simulink library "DYN_2018b"  (Simulink 9.2)
settings: Solver=ode45  StartTime=0.0  StopTime=10.0  RelTol=1e-3  EnableMultiTasking=on
libraries: DYN_AERO x1, DYN_ATT x1, DYN_ECLIPSE x1, DYN_EPHEM x1, DYN_GRAV x1, DYN_MAG x1, DYN_MCI x1, DYN_SRP x1, DYN_TIME x1, DYN_TRA x1
settings Model: Creator=alger  LastModifiedBy=Mike

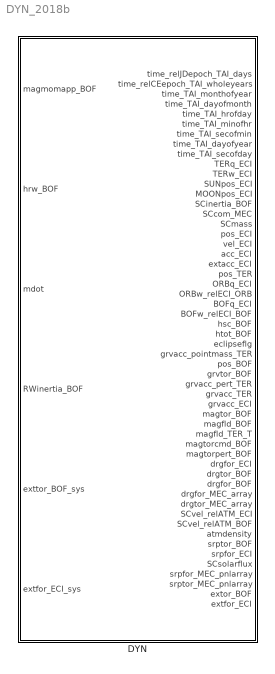
== system DYN_2018b ==
  DYN : Subsystem

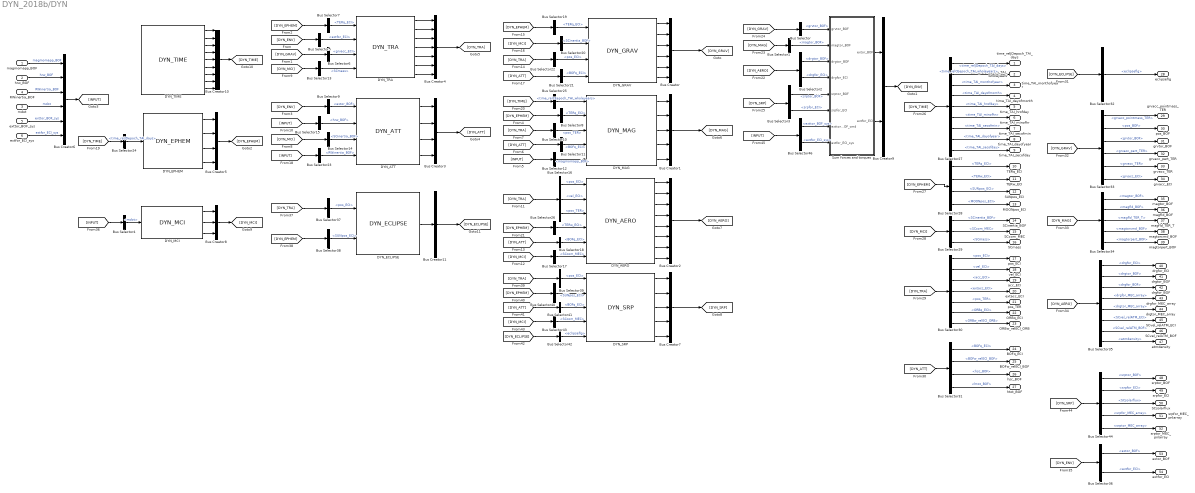
== system DYN_2018b/DYN ==
  magmomapp_BOF : Inport  PortDimensions=3
  hrw_BOF : Inport  Port=2  PortDimensions=3
  mdot : Inport  Port=3  PortDimensions=1
  RWinertia_BOF : Inport  Port=4  PortDimensions=[3,3]
  exttor_BOF_sys : Inport  Port=5  PortDimensions=3
  extfor_ECI_sys : Inport  Port=6  PortDimensions=3
  Bus Creator : BusCreator  Inputs=6
  Bus Creator1 : BusCreator  Inputs=5
  Bus Creator10 : BusCreator  Inputs=9
  Bus Creator11 : BusCreator  Inputs=1
  Bus Creator2 : BusCreator  Inputs=8
  Bus Creator3 : BusCreator  Inputs=4
  Bus Creator4 : BusCreator  Inputs=7
  Bus Creator5 : BusCreator  Inputs=4
  Bus Creator6 : BusCreator  Inputs=6
  Bus Creator7 : BusCreator  Inputs=5
  Bus Creator8 : BusCreator  Inputs=3
  Bus Creator9 : BusCreator  Inputs=2
  Bus Selector : BusSelector  OutputSignals=grvtor_BOF
  Bus Selector1 : BusSelector  OutputSignals=magtor_BOF
  Bus Selector10 : BusSelector  OutputSignals=pos_TER
  Bus Selector{11,18,21,41} (4 alike) : BusSelector  OutputSignals=BOFq_ECI
  Bus Selector12 : BusSelector  OutputSignals=magmomapp_BOF
  Bus Selector13 : BusSelector  OutputSignals=SCmass
  Bus Selector14 : BusSelector  OutputSignals=SCinertia_BOF
  Bus Selector15 : BusSelector  OutputSignals=hrw_BOF
  Bus Selector16 : BusSelector  OutputSignals=pos_ECI,vel_ECI,pos_TER
  Bus Selector17 : BusSelector  OutputSignals=SCcom_MEC
  Bus Selector19 : BusSelector  OutputSignals=TERq_ECI
  Bus Selector2 : BusSelector  OutputSignals=drgtor_BOF,drgfor_ECI
  Bus Selector20 : BusSelector  OutputSignals=SCinertia_BOF
  Bus Selector22 : BusSelector  OutputSignals=pos_ECI
  Bus Selector23 : BusSelector  OutputSignals=RWinertia_BOF
  Bus Selector24 : BusSelector  OutputSignals=time_relJDepoch_TAI_days
  Bus Selector25 : BusSelector  OutputSignals=time_relCEepoch_TAI_wholeyears
  Bus Selector26 : BusSelector  OutputSignals=TERw_ECI
  Bus Selector27 : BusSelector  OutputSignals=time_relJDepoch_TAI_days,time_relCEepoch_TAI_wholeyears,time_TAI_monthofyear,time_TAI_dayofmonth,time_TAI_hrofday,time_TAI_minofhr,time_TAI_secofmin,time_TAI_dayofyear,time_TAI_secofday
  Bus Selector28 : BusSelector  OutputSignals=TERq_ECI,TERw_ECI,SUNpos_ECI,MOONpos_ECI
  Bus Selector29 : BusSelector  OutputSignals=SCinertia_BOF,SCcom_MEC,SCmass
  Bus Selector3 : BusSelector  OutputSignals=srptor_BOF,srpfor_ECI
  Bus Selector30 : BusSelector  OutputSignals=pos_ECI,vel_ECI,acc_ECI,extacc_ECI,pos_TER,ORBq_ECI,ORBw_relECI_ORB
  Bus Selector31 : BusSelector  OutputSignals=BOFq_ECI,BOFw_relECI_BOF,hsc_BOF,htot_BOF
  Bus Selector32 : BusSelector  OutputSignals=eclipseflg
  Bus Selector33 : BusSelector  OutputSignals=grvacc_pointmass_TER,pos_BOF,grvtor_BOF,grvacc_pert_TER,grvacc_TER,grvacc_ECI
  Bus Selector34 : BusSelector  OutputSignals=magtor_BOF,magfld_BOF,magfld_TER_T,magtorcmd_BOF,magtorpert_BOF
  Bus Selector35 : BusSelector  OutputSignals=drgfor_ECI,drgtor_BOF,drgfor_BOF,drgfor_MEC_array,drgtor_MEC_array,SCvel_relATM_ECI,SCvel_relATM_BOF,atmdensity
  Bus Selector36 : BusSelector  OutputSignals=extor_BOF,extfor_ECI
  Bus Selector37 : BusSelector  OutputSignals=pos_ECI
  Bus Selector38 : BusSelector  OutputSignals=SUNpos_ECI
  Bus Selector39 : BusSelector  OutputSignals=pos_ECI
  Bus Selector4 : BusSelector  OutputSignals=mdot
  Bus Selector40 : BusSelector  OutputSignals=SUNpos_ECI
  Bus Selector42 : BusSelector  OutputSignals=eclipseflg
  Bus Selector43 : BusSelector  OutputSignals=SCcom_MEC
  Bus Selector44 : BusSelector  OutputSignals=srptor_BOF,srpfor_ECI,SCsolarflux,srpfor_MEC_array,srptor_MEC_array
  Bus Selector46 : BusSelector  OutputSignals=exttor_BOF_sys,extfor_ECI_sys
  Bus Selector5 : BusSelector  OutputSignals=extfor_ECI
  Bus Selector6 : BusSelector  OutputSignals=grvacc_ECI
  Bus Selector7 : BusSelector  OutputSignals=TERq_ECI
  Bus Selector8 : BusSelector  OutputSignals=TERq_ECI
  Bus Selector9 : BusSelector  OutputSignals=extor_BOF
  DYN_AERO : DYN_AERO/DYN_AERO  SystemSampleTime=-1  Latency=0  AutoFrameSizeCalculation=off
  DYN_ATT : DYN_ATT/DYN_ATT  SystemSampleTime=-1  Latency=0  AutoFrameSizeCalculation=off
  DYN_ECLIPSE : DYN_ECLIPSE/DYN_ECLIPSE  SystemSampleTime=-1  Latency=0  AutoFrameSizeCalculation=off
  DYN_EPHEM : DYN_EPHEM/DYN_EPHEM  SystemSampleTime=-1  Latency=0  AutoFrameSizeCalculation=off
  DYN_GRAV : DYN_GRAV/DYN_GRAV  SystemSampleTime=-1  Latency=0  AutoFrameSizeCalculation=off
  DYN_MAG : DYN_MAG/DYN_MAG  SystemSampleTime=-1  Latency=0  AutoFrameSizeCalculation=off
  DYN_MCI : DYN_MCI/DYN_MCI  SystemSampleTime=-1  Latency=0  AutoFrameSizeCalculation=off
  DYN_SRP : DYN_SRP/DYN_SRP  SystemSampleTime=-1  Latency=0  AutoFrameSizeCalculation=off
  DYN_TIME : DYN_TIME/DYN_TIME  SystemSampleTime=-1  Latency=0  AutoFrameSizeCalculation=off
  "DYN_TRA " : DYN_TRA/DYN_TRA   SystemSampleTime=-1  Latency=0  AutoFrameSizeCalculation=off
  Sum forces and torques : Subsystem
  time_relJDepoch_TAI_days : Outport  VectorParamsAs1DForOutWhenUnconnected=off
  time_relCEepoch_TAI_wholeyears : Outport  Port=2  VectorParamsAs1DForOutWhenUnconnected=off
  time_TAI_monthofyear : Outport  Port=3  VectorParamsAs1DForOutWhenUnconnected=off
  time_TAI_dayofmonth : Outport  Port=4  VectorParamsAs1DForOutWhenUnconnected=off
  time_TAI_hrofday : Outport  Port=5  VectorParamsAs1DForOutWhenUnconnected=off
  time_TAI_minofhr : Outport  Port=6  VectorParamsAs1DForOutWhenUnconnected=off
  time_TAI_secofmin : Outport  Port=7  VectorParamsAs1DForOutWhenUnconnected=off
  time_TAI_dayofyear : Outport  Port=8  VectorParamsAs1DForOutWhenUnconnected=off
  time_TAI_secofday : Outport  Port=9  VectorParamsAs1DForOutWhenUnconnected=off
  TERq_ECI : Outport  Port=10  VectorParamsAs1DForOutWhenUnconnected=off
  TERw_ECI : Outport  Port=11  VectorParamsAs1DForOutWhenUnconnected=off
  SUNpos_ECI : Outport  Port=12  VectorParamsAs1DForOutWhenUnconnected=off
  MOONpos_ECI : Outport  Port=13  VectorParamsAs1DForOutWhenUnconnected=off
  SCinertia_BOF : Outport  Port=14  VectorParamsAs1DForOutWhenUnconnected=off
  SCcom_MEC : Outport  Port=15  VectorParamsAs1DForOutWhenUnconnected=off
  SCmass : Outport  Port=16  VectorParamsAs1DForOutWhenUnconnected=off
  pos_ECI : Outport  Port=17  VectorParamsAs1DForOutWhenUnconnected=off
  vel_ECI : Outport  Port=18  VectorParamsAs1DForOutWhenUnconnected=off
  acc_ECI : Outport  Port=19  VectorParamsAs1DForOutWhenUnconnected=off
  extacc_ECI : Outport  Port=20  VectorParamsAs1DForOutWhenUnconnected=off
  pos_TER : Outport  Port=21  VectorParamsAs1DForOutWhenUnconnected=off
  ORBq_ECI : Outport  Port=22  VectorParamsAs1DForOutWhenUnconnected=off
  ORBw_relECI_ORB : Outport  Port=23  PortDimensions=3  VectorParamsAs1DForOutWhenUnconnected=off
  BOFq_ECI : Outport  Port=24  VectorParamsAs1DForOutWhenUnconnected=off
  BOFw_relECI_BOF : Outport  Port=25  VectorParamsAs1DForOutWhenUnconnected=off
  hsc_BOF : Outport  Port=26  VectorParamsAs1DForOutWhenUnconnected=off
  htot_BOF : Outport  Port=27  VectorParamsAs1DForOutWhenUnconnected=off
  eclipseflg : Outport  Port=28  VectorParamsAs1DForOutWhenUnconnected=off
  grvacc_pointmass_TER : Outport  Port=29  VectorParamsAs1DForOutWhenUnconnected=off
  pos_BOF : Outport  Port=30  VectorParamsAs1DForOutWhenUnconnected=off
  grvtor_BOF : Outport  Port=31  VectorParamsAs1DForOutWhenUnconnected=off
  grvacc_pert_TER : Outport  Port=32  VectorParamsAs1DForOutWhenUnconnected=off
  grvacc_TER : Outport  Port=33  VectorParamsAs1DForOutWhenUnconnected=off
  grvacc_ECI : Outport  Port=34  VectorParamsAs1DForOutWhenUnconnected=off
  magtor_BOF : Outport  Port=35  VectorParamsAs1DForOutWhenUnconnected=off
  magfld_BOF : Outport  Port=36  VectorParamsAs1DForOutWhenUnconnected=off
  magfld_TER_T : Outport  Port=37  VectorParamsAs1DForOutWhenUnconnected=off
  magtorcmd_BOF : Outport  Port=38  VectorParamsAs1DForOutWhenUnconnected=off
  magtorpert_BOF : Outport  Port=39  VectorParamsAs1DForOutWhenUnconnected=off
  drgfor_ECI : Outport  Port=40  VectorParamsAs1DForOutWhenUnconnected=off
  drgtor_BOF : Outport  Port=41  VectorParamsAs1DForOutWhenUnconnected=off
  drgfor_BOF : Outport  Port=42  VectorParamsAs1DForOutWhenUnconnected=off
  drgfor_MEC_array : Outport  Port=43  VectorParamsAs1DForOutWhenUnconnected=off
  drgtor_MEC_array : Outport  Port=44  VectorParamsAs1DForOutWhenUnconnected=off
  SCvel_relATM_ECI : Outport  Port=45  VectorParamsAs1DForOutWhenUnconnected=off
  SCvel_relATM_BOF : Outport  Port=46  VectorParamsAs1DForOutWhenUnconnected=off
  atmdensity : Outport  Port=47  VectorParamsAs1DForOutWhenUnconnected=off
  srptor_BOF : Outport  Port=48  PortDimensions=3  VectorParamsAs1DForOutWhenUnconnected=off
  srpfor_ECI : Outport  Port=49  PortDimensions=3  VectorParamsAs1DForOutWhenUnconnected=off
  SCsolarflux : Outport  Port=50  VectorParamsAs1DForOutWhenUnconnected=off
  srpfor_MEC_pnlarray : Outport  Port=51  VectorParamsAs1DForOutWhenUnconnected=off
  srptor_MEC_pnlarray : Outport  Port=52  VectorParamsAs1DForOutWhenUnconnected=off
  extor_BOF : Outport  Port=53  VectorParamsAs1DForOutWhenUnconnected=off
  extfor_ECI : Outport  Port=54  VectorParamsAs1DForOutWhenUnconnected=off
  wires:
  magmomapp_BOF/1 -> Bus Creator6/1  "magmomapp_BOF"
  DYN_MAG/2 -> Bus Creator1/2
  DYN_MAG/1 -> Bus Creator1/1
  DYN_MAG/3 -> Bus Creator1/3
  DYN_GRAV/2 -> Bus Creator/2
  DYN_GRAV/1 -> Bus Creator/1
  DYN_GRAV/3 -> Bus Creator/3
  DYN_GRAV/4 -> Bus Creator/4
  DYN_GRAV/5 -> Bus Creator/5
  DYN_GRAV/6 -> Bus Creator/6
  DYN_AERO/3 -> Bus Creator2/3
  DYN_AERO/4 -> Bus Creator2/4
  DYN_AERO/2 -> Bus Creator2/2
  DYN_AERO/5 -> Bus Creator2/5
  DYN_AERO/1 -> Bus Creator2/1
  DYN_AERO/6 -> Bus Creator2/6
  DYN_AERO/7 -> Bus Creator2/7
  DYN_AERO/8 -> Bus Creator2/8
  DYN_ATT/1 -> Bus Creator3/1
  DYN_ATT/2 -> Bus Creator3/2
  DYN_ATT/3 -> Bus Creator3/3
  DYN_ATT/4 -> Bus Creator3/4
  "DYN_TRA "/2 -> Bus Creator4/2
  "DYN_TRA "/4 -> Bus Creator4/4
  "DYN_TRA "/1 -> Bus Creator4/1
  "DYN_TRA "/3 -> Bus Creator4/3
  "DYN_TRA "/5 -> Bus Creator4/5
  DYN_EPHEM/3 -> Bus Creator5/3
  DYN_EPHEM/2 -> Bus Creator5/2
  DYN_EPHEM/4 -> Bus Creator5/4
  DYN_EPHEM/1 -> Bus Creator5/1
  Bus Creator1/1 -> [DYN_MAG]
  Bus Creator2/1 -> [DYN_AERO]
  DYN_SRP/2 -> Bus Creator7/2
  DYN_SRP/1 -> Bus Creator7/1
  Bus Creator7/1 -> [DYN_SRP]
  hrw_BOF/1 -> Bus Creator6/2  "hrw_BOF"
  mdot/1 -> Bus Creator6/4  "mdot"
  DYN_MCI/1 -> Bus Creator8/1
  DYN_MCI/2 -> Bus Creator8/2
  DYN_MCI/3 -> Bus Creator8/3
  Bus Selector4/1 -> DYN_MCI/1  "<mdot>"
  Bus Creator6/1 -> [INPUT]
  Bus Selector/1 -> Sum forces and torques/1(grvtor_BOF)  "<grvtor_BOF>"
  Bus Selector1/1 -> Sum forces and torques/2(magtor_BOF)  "<magtor_BOF>"
  Bus Selector2/1 -> Sum forces and torques/3(drgtor_BOF)  "<drgtor_BOF>"
  Bus Selector2/2 -> Sum forces and torques/4(drgfor_ECI)  "<drgfor_ECI>"
  Bus Selector3/1 -> Sum forces and torques/5(srptor_BOF)  "<srptor_BOF>"
  Bus Selector3/2 -> Sum forces and torques/6(srpfor_ECI)  "<srpfor_ECI>"
  Sum forces and torques/1(extor_BOF) -> Bus Creator9/1
  Sum forces and torques/2(extfor_ECI) -> Bus Creator9/2
  Bus Selector6/1 -> "DYN_TRA "/3  "<grvacc_ECI>"
  Bus Creator/1 -> [DYN_GRAV]
  Bus Selector5/1 -> "DYN_TRA "/2  "<extfor_ECI>"
  Bus Selector7/1 -> "DYN_TRA "/1  "<TERq_ECI>"
  [DYN_GRAV] -> Bus Selector6/1
  Bus Creator9/1 -> [DYN_ENV]
  [DYN_ENV] -> Bus Selector5/1
  [DYN_EPHEM] -> Bus Selector7/1
  Bus Creator5/1 -> [DYN_EPHEM]
  Bus Selector8/1 -> DYN_MAG/2  "<TERq_ECI>"
  [DYN_EPHEM] -> Bus Selector8/1
  Bus Selector10/1 -> DYN_MAG/3  "<pos_TER>"
  Bus Creator4/1 -> [DYN_TRA]
  Bus Selector11/1 -> DYN_MAG/4  "<BOFq_ECI>"
  Bus Creator3/1 -> [DYN_ATT]
  Bus Selector9/1 -> DYN_ATT/1  "<extor_BOF>"
  [DYN_ENV] -> Bus Selector9/1
  [DYN_ATT] -> Bus Selector11/1
  [INPUT] -> Bus Selector12/1
  Bus Selector12/1 -> DYN_MAG/5  "<magmomapp_BOF>"
  [DYN_TRA] -> Bus Selector10/1
  Bus Creator8/1 -> [DYN_MCI]
  [DYN_MCI] -> Bus Selector13/1
  [DYN_MCI] -> Bus Selector14/1
  Bus Selector14/1 -> DYN_ATT/3  "<SCinertia_BOF>"
  [INPUT] -> Bus Selector15/1
  Bus Selector15/1 -> DYN_ATT/2  "<hrw_BOF>"
  RWinertia_BOF/1 -> Bus Creator6/3  "RWinertia_BOF"
  [DYN_TRA] -> Bus Selector16/1
  Bus Selector16/1 -> DYN_AERO/1  "<pos_ECI>"
  Bus Selector16/2 -> DYN_AERO/2  "<vel_ECI>"
  Bus Selector16/3 -> DYN_AERO/3  "<pos_TER>"
  [DYN_MCI] -> Bus Selector17/1
  Bus Selector17/1 -> DYN_AERO/6  "<SCcom_MEC>"
  [DYN_ATT] -> Bus Selector18/1
  Bus Selector13/1 -> "DYN_TRA "/4  "<SCmass>"
  [DYN_EPHEM] -> Bus Selector19/1
  Bus Selector19/1 -> DYN_GRAV/1  "<TERq_ECI>"
  [DYN_MCI] -> Bus Selector20/1
  Bus Selector20/1 -> DYN_GRAV/2  "<SCinertia_BOF>"
  [DYN_ATT] -> Bus Selector21/1
  [DYN_TRA] -> Bus Selector22/1
  Bus Selector22/1 -> DYN_GRAV/3  "<pos_ECI>"
  Bus Selector21/1 -> DYN_GRAV/4  "<BOFq_ECI>"
  [INPUT] -> Bus Selector23/1
  Bus Selector23/1 -> DYN_ATT/4  "<RWinertia_BOF>"
  DYN_TIME/1 -> Bus Creator10/1
  Bus Selector24/1 -> DYN_EPHEM/1  "<time_relJDepoch_TAI_days>"
  [DYN_TIME] -> Bus Selector24/1
  Bus Creator10/1 -> [DYN_TIME]
  DYN_TIME/9 -> Bus Creator10/9
  DYN_TIME/8 -> Bus Creator10/8
  DYN_TIME/5 -> Bus Creator10/5
  DYN_TIME/3 -> Bus Creator10/3
  DYN_TIME/6 -> Bus Creator10/6
  DYN_TIME/7 -> Bus Creator10/7
  DYN_TIME/2 -> Bus Creator10/2
  DYN_TIME/4 -> Bus Creator10/4
  Bus Selector25/1 -> DYN_MAG/1  "<time_relCEepoch_TAI_wholeyears>"
  [DYN_TIME] -> Bus Selector25/1
  Bus Selector18/1 -> DYN_AERO/5  "<BOFq_ECI>"
  Bus Selector26/1 -> DYN_AERO/4  "<TERw_ECI>"
  [DYN_EPHEM] -> Bus Selector26/1
  [DYN_AERO] -> Bus Selector2/1
  [DYN_MAG] -> Bus Selector1/1
  [DYN_GRAV] -> Bus Selector/1
  [DYN_SRP] -> Bus Selector3/1
  Bus Creator11/1 -> [DYN_ECLIPSE]
  DYN_ECLIPSE/1 -> Bus Creator11/1
  [DYN_TIME] -> Bus Selector27/1
  [DYN_EPHEM] -> Bus Selector28/1
  [DYN_MCI] -> Bus Selector29/1
  [DYN_TRA] -> Bus Selector30/1
  Bus Selector27/1 -> time_relJDepoch_TAI_days/1  "<time_relJDepoch_TAI_days>"
  Bus Selector27/2 -> time_relCEepoch_TAI_wholeyears/1  "<time_relCEepoch_TAI_wholeyears>"
  Bus Selector27/3 -> time_TAI_monthofyear/1  "<time_TAI_monthofyear>"
  Bus Selector27/4 -> time_TAI_dayofmonth/1  "<time_TAI_dayofmonth>"
  Bus Selector27/5 -> time_TAI_hrofday/1  "<time_TAI_hrofday>"
  Bus Selector27/6 -> time_TAI_minofhr/1  "<time_TAI_minofhr>"
  Bus Selector27/7 -> time_TAI_secofmin/1  "<time_TAI_secofmin>"
  Bus Selector27/8 -> time_TAI_dayofyear/1  "<time_TAI_dayofyear>"
  Bus Selector27/9 -> time_TAI_secofday/1  "<time_TAI_secofday>"
  Bus Selector28/1 -> TERq_ECI/1  "<TERq_ECI>"
  Bus Selector28/4 -> MOONpos_ECI/1  "<MOONpos_ECI>"
  Bus Selector28/3 -> SUNpos_ECI/1  "<SUNpos_ECI>"
  Bus Selector28/2 -> TERw_ECI/1  "<TERw_ECI>"
  Bus Selector29/1 -> SCinertia_BOF/1  "<SCinertia_BOF>"
  Bus Selector29/2 -> SCcom_MEC/1  "<SCcom_MEC>"
  Bus Selector29/3 -> SCmass/1  "<SCmass>"
  [INPUT] -> Bus Selector4/1
  Bus Selector30/5 -> pos_TER/1  "<pos_TER>"
  Bus Selector30/1 -> pos_ECI/1  "<pos_ECI>"
  Bus Selector30/2 -> vel_ECI/1  "<vel_ECI>"
  Bus Selector30/3 -> acc_ECI/1  "<acc_ECI>"
  Bus Selector30/4 -> extacc_ECI/1  "<extacc_ECI>"
  [DYN_ATT] -> Bus Selector31/1
  Bus Selector31/4 -> htot_BOF/1  "<htot_BOF>"
  Bus Selector31/1 -> BOFq_ECI/1  "<BOFq_ECI>"
  Bus Selector31/2 -> BOFw_relECI_BOF/1  "<BOFw_relECI_BOF>"
  Bus Selector31/3 -> hsc_BOF/1  "<hsc_BOF>"
  Bus Selector37/1 -> DYN_ECLIPSE/1  "<pos_ECI>"
  [DYN_ECLIPSE] -> Bus Selector32/1
  Bus Selector32/1 -> eclipseflg/1  "<eclipseflg>"
  [DYN_GRAV] -> Bus Selector33/1
  Bus Selector33/1 -> grvacc_pointmass_TER/1  "<grvacc_pointmass_TER>"
  Bus Selector33/2 -> pos_BOF/1  "<pos_BOF>"
  Bus Selector33/3 -> grvtor_BOF/1  "<grvtor_BOF>"
  Bus Selector33/4 -> grvacc_pert_TER/1  "<grvacc_pert_TER>"
  Bus Selector33/5 -> grvacc_TER/1  "<grvacc_TER>"
  Bus Selector33/6 -> grvacc_ECI/1  "<grvacc_ECI>"
  [DYN_MAG] -> Bus Selector34/1
  [DYN_AERO] -> Bus Selector35/1
  Bus Selector34/1 -> magtor_BOF/1  "<magtor_BOF>"
  Bus Selector34/2 -> magfld_BOF/1  "<magfld_BOF>"
  Bus Selector34/3 -> magfld_TER_T/1  "<magfld_TER_T>"
  Bus Selector35/1 -> drgfor_ECI/1  "<drgfor_ECI>"
  Bus Selector35/2 -> drgtor_BOF/1  "<drgtor_BOF>"
  Bus Selector35/3 -> drgfor_BOF/1  "<drgfor_BOF>"
  Bus Selector35/4 -> drgfor_MEC_array/1  "<drgfor_MEC_array>"
  Bus Selector35/5 -> drgtor_MEC_array/1  "<drgtor_MEC_array>"
  Bus Selector35/6 -> SCvel_relATM_ECI/1  "<SCvel_relATM_ECI>"
  Bus Selector35/7 -> SCvel_relATM_BOF/1  "<SCvel_relATM_BOF>"
  Bus Selector35/8 -> atmdensity/1  "<atmdensity>"
  [DYN_ENV] -> Bus Selector36/1
  Bus Selector36/2 -> extfor_ECI/1  "<extfor_ECI>"
  Bus Selector36/1 -> extor_BOF/1  "<extor_BOF>"
  DYN_MAG/4 -> Bus Creator1/4
  DYN_MAG/5 -> Bus Creator1/5
  Bus Selector34/4 -> magtorcmd_BOF/1  "<magtorcmd_BOF>"
  Bus Selector34/5 -> magtorpert_BOF/1  "<magtorpert_BOF>"
  "DYN_TRA "/6 -> Bus Creator4/6
  Bus Selector30/6 -> ORBq_ECI/1  "<ORBq_ECI>"
  [DYN_TRA] -> Bus Selector37/1
  Bus Selector38/1 -> DYN_ECLIPSE/2  "<SUNpos_ECI>"
  [DYN_EPHEM] -> Bus Selector38/1
  Bus Selector39/1 -> DYN_SRP/1  "<pos_ECI>"
  [DYN_TRA] -> Bus Selector39/1
  Bus Selector40/1 -> DYN_SRP/2  "<SUNpos_ECI>"
  [DYN_EPHEM] -> Bus Selector40/1
  [DYN_ATT] -> Bus Selector41/1
  Bus Selector41/1 -> DYN_SRP/3  "<BOFq_ECI>"
  DYN_SRP/3 -> Bus Creator7/3
  [DYN_ECLIPSE] -> Bus Selector42/1
  Bus Selector42/1 -> DYN_SRP/5  "<eclipseflg>"
  [DYN_MCI] -> Bus Selector43/1
  Bus Selector43/1 -> DYN_SRP/4  "<SCcom_MEC>"
  DYN_SRP/4 -> Bus Creator7/4
  DYN_SRP/5 -> Bus Creator7/5
  [DYN_SRP] -> Bus Selector44/1
  Bus Selector44/1 -> srptor_BOF/1  "<srptor_BOF>"
  Bus Selector44/2 -> srpfor_ECI/1  "<srpfor_ECI>"
  Bus Selector44/3 -> SCsolarflux/1  "<SCsolarflux>"
  Bus Selector44/4 -> srpfor_MEC_pnlarray/1  "<srpfor_MEC_array>"
  Bus Selector44/5 -> srptor_MEC_pnlarray/1  "<srptor_MEC_array>"
  exttor_BOF_sys/1 -> Bus Creator6/5  "exttor_BOF_sys"
  extfor_ECI_sys/1 -> Bus Creator6/6  "extfor_ECI_sys"
  [INPUT] -> Bus Selector46/1
  Bus Selector46/1 -> Sum forces and torques/7(exttor_BOF_cmd)  "<exttor_BOF_sys>"
  Bus Selector46/2 -> Sum forces and torques/8(extfor_ECI_sys)  "<extfor_ECI_sys>"
  "DYN_TRA "/7 -> Bus Creator4/7
  Bus Selector30/7 -> ORBw_relECI_ORB/1  "<ORBw_relECI_ORB>"

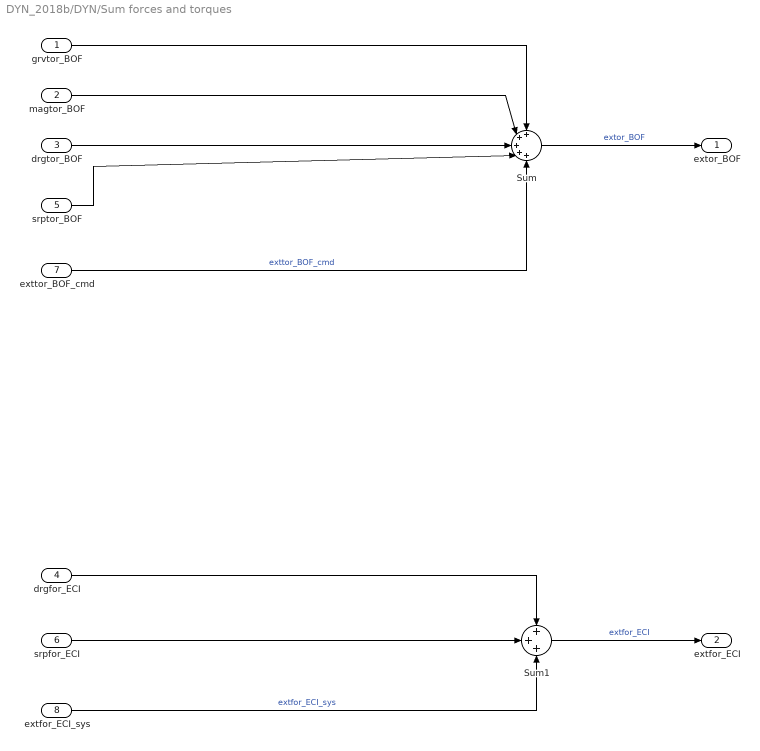
== system DYN_2018b/DYN/Sum forces and torques ==
  grvtor_BOF : Inport
  magtor_BOF : Inport  Port=2
  drgtor_BOF : Inport  Port=3
  drgfor_ECI : Inport  Port=4
  srptor_BOF : Inport  Port=5
  srpfor_ECI : Inport  Port=6
  exttor_BOF_cmd : Inport  Port=7  PortDimensions=3
  extfor_ECI_sys : Inport  Port=8  PortDimensions=3
  Sum : Sum  Inputs=+++++
  Sum1 : Sum  Inputs=+++
  extor_BOF : Outport  VectorParamsAs1DForOutWhenUnconnected=off
  extfor_ECI : Outport  Port=2  VectorParamsAs1DForOutWhenUnconnected=off
  wires:
  Sum1/1 -> extfor_ECI/1  "extfor_ECI"
  Sum/1 -> extor_BOF/1  "extor_BOF"
  drgtor_BOF/1 -> Sum/3
  srptor_BOF/1 -> Sum/4
  magtor_BOF/1 -> Sum/2
  grvtor_BOF/1 -> Sum/1
  drgfor_ECI/1 -> Sum1/1
  srpfor_ECI/1 -> Sum1/2
  exttor_BOF_cmd/1 -> Sum/5  "exttor_BOF_cmd"
  extfor_ECI_sys/1 -> Sum1/3  "extfor_ECI_sys"
